simulink library "dsrc_util_lib"  (Simulink 8.2)
settings: Solver=ode1  StartTime=0.0  StopTime=Inf  FixedStep=0.001  RelTol=1e-3
PostLoadFcn:
  | , if any(exist('dsrtsu_mdlpostloadfcn', 'file') == [2, 3, 6]), try dsrtsu_mdlpostloadfcn('Execute', bdroot); catch fprintf('Error in PostLoadFcn (dsrtsu_mdlpostloadfcn) for model "%s":\n %s\n', bdroot, lasterr); end, end,
settings Model: DSRTSU_INTERNAL_RTI_VER=450  DSRTSU_INTERNAL_RTI_TYPE=rti1401  DSRTSU_INTERNAL_RTIFPGA=40  Creator=rushk1  LastModifiedBy=rushk1

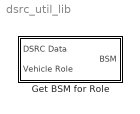
== system dsrc_util_lib ==
  Get BSM for Role : Subsystem

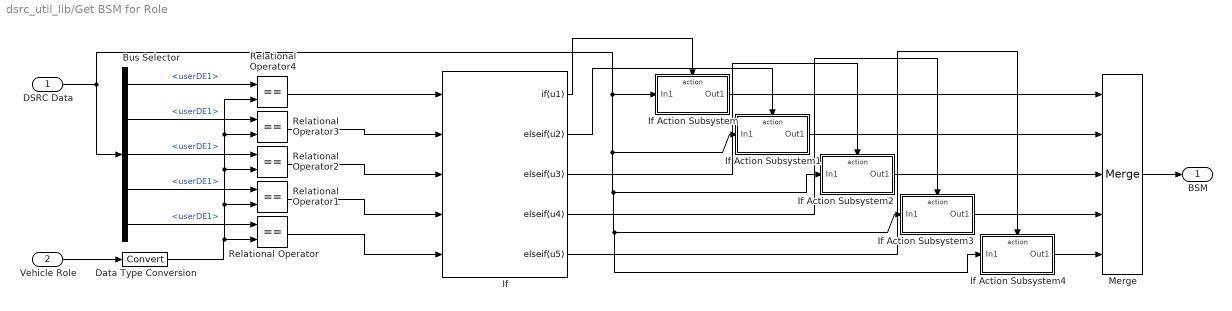
== system dsrc_util_lib/Get BSM for Role ==
  DSRC Data : Inport  OutDataTypeStr=Bus: BSMStoreBus
  Vehicle Role : Inport  Port=2  OutDataTypeStr=Enum: VehicleRoleEnum
  Bus Selector : BusSelector  OutputSignals=Veh1BSM.userDE1,Veh2BSM.userDE1,Veh3BSM.userDE1,Veh4BSM.userDE1,Veh5BSM.userDE1
  Data Type Conversion : DataTypeConversion
  If : If  NumInputs=5  IfExpression=u1  ElseIfExpressions=u2,u3, u4, u5  ShowElse=off
  If Action Subsystem : Subsystem  TreatAsAtomicUnit=on
  If Action Subsystem1 : Subsystem  TreatAsAtomicUnit=on
  If Action Subsystem2 : Subsystem  TreatAsAtomicUnit=on
  If Action Subsystem3 : Subsystem  TreatAsAtomicUnit=on
  If Action Subsystem4 : Subsystem  TreatAsAtomicUnit=on
  Merge : Merge  Inputs=5
  Relational Operator{,1..4} (5 alike) : RelationalOperator  Operator===  OutDataTypeStr=boolean
  BSM : Outport
  wires:
  DSRC Data/1 -> Bus Selector/1, If Action Subsystem4/1(In1), If Action Subsystem3/1(In1), If Action Subsystem2/1(In1), If Action Subsystem1/1(In1), If Action Subsystem/1(In1)
  If/1 -> If Action Subsystem/Action
  If/2 -> If Action Subsystem1/Action
  If/3 -> If Action Subsystem2/Action
  If/4 -> If Action Subsystem3/Action
  If/5 -> If Action Subsystem4/Action
  If Action Subsystem4/1(Out1) -> Merge/5
  If Action Subsystem3/1(Out1) -> Merge/4
  If Action Subsystem2/1(Out1) -> Merge/3
  If Action Subsystem1/1(Out1) -> Merge/2
  If Action Subsystem/1(Out1) -> Merge/1
  Merge/1 -> BSM/1
  Bus Selector/5 -> Relational Operator/1  "<userDE1>"
  Relational Operator/1 -> If/5
  Vehicle Role/1 -> Data Type Conversion/1
  Bus Selector/4 -> Relational Operator1/1  "<userDE1>"
  Relational Operator1/1 -> If/4
  Bus Selector/3 -> Relational Operator2/1  "<userDE1>"
  Relational Operator2/1 -> If/3
  Bus Selector/2 -> Relational Operator3/1  "<userDE1>"
  Relational Operator3/1 -> If/2
  Bus Selector/1 -> Relational Operator4/1  "<userDE1>"
  Relational Operator4/1 -> If/1
  Data Type Conversion/1 -> Relational Operator4/2, Relational Operator3/2, Relational Operator2/2, Relational Operator1/2, Relational Operator/2

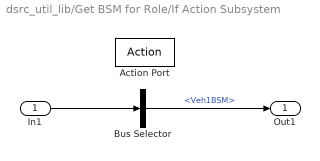
== system dsrc_util_lib/Get BSM for Role/If Action Subsystem ==
  In1 : Inport
  Action Port : ActionPort
  Bus Selector : BusSelector  OutputSignals=Veh1BSM
  Out1 : Outport
  wires:
  In1/1 -> Bus Selector/1
  Bus Selector/1 -> Out1/1  "<Veh1BSM>"

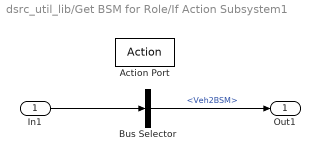
== system dsrc_util_lib/Get BSM for Role/If Action Subsystem1 ==
  In1 : Inport
  Action Port : ActionPort
  Bus Selector : BusSelector  OutputSignals=Veh2BSM
  Out1 : Outport
  wires:
  In1/1 -> Bus Selector/1
  Bus Selector/1 -> Out1/1  "<Veh2BSM>"

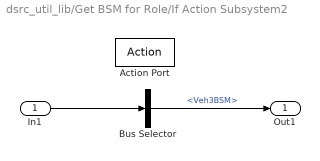
== system dsrc_util_lib/Get BSM for Role/If Action Subsystem2 ==
  In1 : Inport
  Action Port : ActionPort
  Bus Selector : BusSelector  OutputSignals=Veh3BSM
  Out1 : Outport
  wires:
  In1/1 -> Bus Selector/1
  Bus Selector/1 -> Out1/1  "<Veh3BSM>"

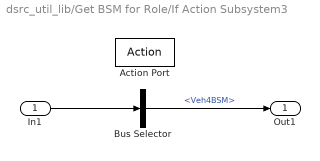
== system dsrc_util_lib/Get BSM for Role/If Action Subsystem3 ==
  In1 : Inport
  Action Port : ActionPort
  Bus Selector : BusSelector  OutputSignals=Veh4BSM
  Out1 : Outport
  wires:
  In1/1 -> Bus Selector/1
  Bus Selector/1 -> Out1/1  "<Veh4BSM>"

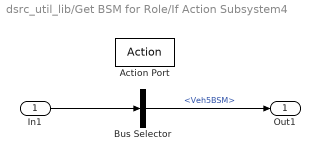
== system dsrc_util_lib/Get BSM for Role/If Action Subsystem4 ==
  In1 : Inport
  Action Port : ActionPort
  Bus Selector : BusSelector  OutputSignals=Veh5BSM
  Out1 : Outport
  wires:
  In1/1 -> Bus Selector/1
  Bus Selector/1 -> Out1/1  "<Veh5BSM>"
